simulink model "SimplifiedThreeDOFModel"  (R2022b)
settings: Solver=VariableStepAuto  StartTime=0.0  StopTime=10.0  RelTol=1e-3
values from neighbouring files (symbols this model uses):
  omega = 90    [ThreeDOF.m]
undefined symbols (not defined in the file or in its folder): r, v
libraries: simulink x2
settings Model: Creator=ruben  LastModifiedBy=ruben

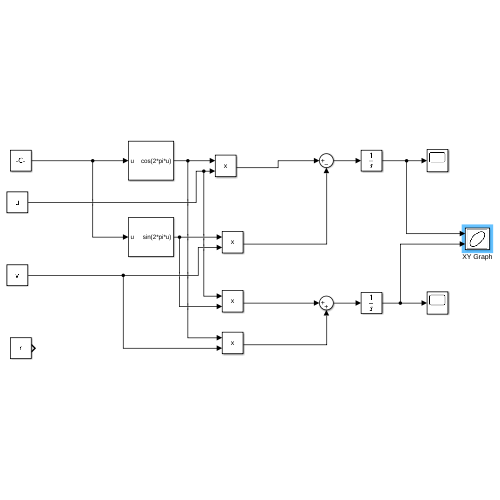
[thumbnail: Simulink's stored preview of the top-level diagram]
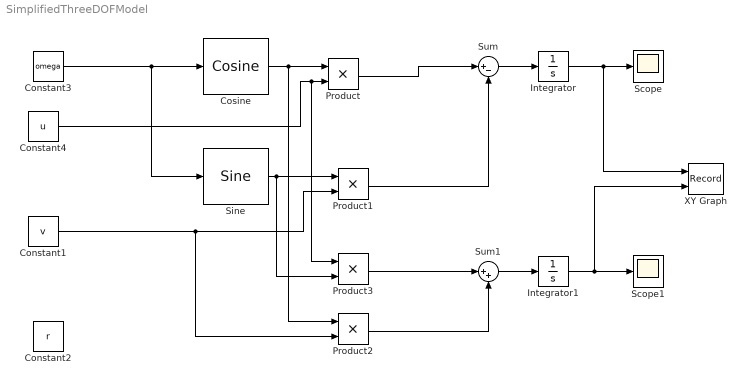
== system SimplifiedThreeDOFModel ==
  Constant1 : Constant  Value=v
  Constant2 : Constant  Value=r
  Constant3 : Constant  Value=omega
  Constant4 : Constant  Value=u
  Cosine : simulink/Lookup Tables/Cosine  Formula=cos(2*pi*u)  NumDataPoints=(2^5)+1  OutputWordLength=16  InternalRulePriority=Speed
  Integrator : Integrator
  Integrator1 : Integrator
  Product{,1..3} (4 alike) : Product
  Scope : Scope
  Scope1 : Scope
  Sine : simulink/Lookup Tables/Sine  Formula=sin(2*pi*u)  NumDataPoints=(2^5)+1  OutputWordLength=16  InternalRulePriority=Speed
  Sum : Sum  Inputs=|+-
  Sum1 : Sum  Inputs=|++
  XY Graph : Record  FileSettingsInternal="{\"entries\":[{\"content\":{\"excelSettings\":{\"content\":{},\"type\":\"Streamout.ExcelSettings\"}},\"type\":\"Streamout.FileSettingStorage\",\"uuid\":\"3ece6f28-7960-4ee8-836b-1968017b9ec3\"}],\"packageUris\":[\"http://schema.mathworks.com/mf0/streamout_blocks/R2020a\"],\"version\":\"1.0\"}"  Layout=[1 1]  SignalsInternal="{\"entries\":[{\"content\":{\"signals\":[{\"content\":{\"blockPath\":[\"untitled/XY Graph\"],\"channel\":[],\"dimensions\":[1],\"domain\":\"untitled/XY Graph\",\"lineColor\":\"#a2142f\",\"plots\":[1],\"port\":1,\"sid\":[\"\"],\"signalID\":129,\"signalName\":\"Integrator\"},\"type\":\"RecordBlkView.Signal\",\"uuid\":\"8d8a1a15-49ad-418f-8601-77fd79409db0\"},{\"content\":{\"blockPath\":[\"untitled/XY Graph\"],\"channel\":[],\"dimensions\":[1],\"domain\":\"untitled/XY Graph\",\"lineColor\":\"#139fff\",\"plots\":[1],\"port\":2,\"sid\":[\"\"],\"signalID\":133,\"signalName\":\"Integrator1\"},\"type\":\"RecordBlkView.Signal\",\"uuid\":\"8f5b13d7-87d5-4c13-8064-4511b103dad9\"}]},\"type\":\"RecordBlkView.InputSignals\",\"uuid\":\"bf495e5f-cca6-4887-b79a-235ea3ea4fc6\"}],\"packageUris\":[\"http://schema.mathworks.com/mf0/streamout_blocks/R2020a\"],\"version\":\"1.0\"}"  VisualizationBindings="{\"xyplotplugin\":{\"info\":[{\"series\":[{\"bindingParametersList\":[{\"parameter\":\"X-Axis\",\"signalID\":129,\"signalName\":\"Integrator\"},{\"parameter\":\"Y-Axis\",\"signalID\":133,\"signalName\":\"Integrator1\"}],\"seriesID\":21828}],\"subplotID\":1}]}}"  CompatibilityTag=XY
  wires:
  Constant3/1 -> Sine/1, Cosine/1
  Cosine/1 -> Product2/1, Product/1
  Constant4/1 -> Product3/1, Product/2
  Product/1 -> Sum/1
  Sine/1 -> Product3/2, Product1/1
  Constant1/1 -> Product2/2, Product1/2
  Product1/1 -> Sum/2
  Product3/1 -> Sum1/1
  Product2/1 -> Sum1/2
  Sum/1 -> Integrator/1
  Sum1/1 -> Integrator1/1
  Integrator1/1 -> XY Graph/2, Scope1/1
  Integrator/1 -> XY Graph/1, Scope/1
